simulink model "sampling_SH_lowpass_sinusoidal"  (R2020a)
settings: Solver=ode45  StartTime=0  StopTime=0.0504045  RelTol=1e-3  EnableMultiTasking=on
PreLoadFcn:
  | seed=123456789;
  | fs=100000;
libraries: dsparch4 x1, dspsigops x1
settings Model: Creator=morelos_zaragoza  LastModifiedBy=000098944
settings DataIOCC: LimitDataPoints=on  SaveFormat=Array  SignalLoggingSaveFormat=ModelDataLogs  ReturnWorkspaceOutputs=off
settings OptimizationCC: ExpressionDepthLimit=2147483647  InitFltsAndDblsToZero=on  LifeSpan=inf
settings DebuggingCC: SaveWithParameterizedLinksMsg=none  UnderspecifiedInitializationDetection=Classic  MergeDetectMultiDrivingBlocksExec=none  SignalResolutionControl=TryResolveAllWithWarning  SolverPrmCheckMsg=warning  MultiTaskDSMMsg=warning  MultiTaskCondExecSysMsg=none  FcnCallInpInsideContextMsg=warning  StateNameClashWarn=warning  SFUnexpectedBacktrackingDiag=warning  SFNoUnconditionalDefaultTransitionDiag=warning  SFExecutionAtInitializationDiag=none  ArithmeticOperatorsInVariantConditions=warning
settings HardwareCC: ProdBitPerPointer=32  ProdBitPerSizeT=32  ProdBitPerPtrDiffT=32  ProdLargestAtomicFloat=None  ProdIntDivRoundTo=Undefined  ProdEndianess=Unspecified  ProdWordSize=32  ProdHWDeviceType=32-bit Generic
settings ModelReferenceCC: PropagateSignalLabelsOutOfModel=off
settings SFSimCC: SimUseLocalCustomCode=off  CustomCodeUndefinedFunction=UseInterfaceOnly
settings RTWCC: RTWUseLocalCustomCode=off
settings CodeAppCC: StateflowObjectComments=on
settings GRTTargetCC: TargetFcnLib=ansi_tfl_tmw.mat  TargetLangStandard=C89/C90 (ANSI)  CombineOutputUpdateFcns=off  GRTInterface=on
settings ConfigComp: CovMetricSettings=dw  CovHtmlReporting=on  CovSaveCumulativeToWorkspaceVar=on  CovSaveSingleToWorkspaceVar=on  CovExternalEMLEnable=off

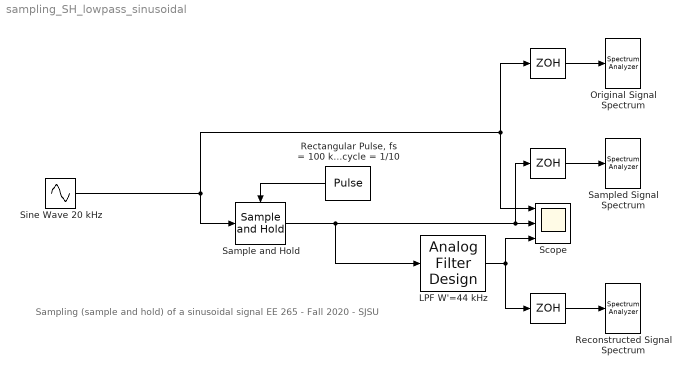
== system sampling_SH_lowpass_sinusoidal ==
  note: Sampling (sample and hold) of a sinusoidal signal
      | EE 265 - Fall 2020 - SJSU
  "  " : ZeroOrderHold  SampleTime=1/600000
  "    " : ZeroOrderHold  SampleTime=1/600000
  "     " : ZeroOrderHold  SampleTime=1/600000
  " Original Signal Spectrum" : SpectrumAnalyzer
  LPF W'=44 kHz : dsparch4/Analog Filter Design  method=Butterworth  filttype=Lowpass  N=8  Wlo=2*pi*44000  Whi=2*pi*110  Rp=2  Rs=40
  Reconstructed Signal Spectrum : SpectrumAnalyzer
  "Rectangular Pulse, fs = 100 kHz Duty cycle = 1/10" : DiscretePulseGenerator  PulseType=Time based  Period=1/fs  PulseWidth=10  SampleTime=1e-2/2)
  Sample and Hold : dspsigops/Sample and Hold  trig=Rising edge  initCond=0  latchinput=off
  Sampled Signal Spectrum : SpectrumAnalyzer
  Scope : Scope  NumInputPorts=3
  Sine Wave 20 kHz : Sin  Frequency=2*pi*20000  Phase=pi/6  SampleTime=0
  wires:
  Sample and Hold/1 -> LPF W'=44 kHz/1, "  "/1, Scope/2
  "  "/1 -> Sampled Signal Spectrum/1
  Sine Wave 20 kHz/1 -> Sample and Hold/1, "     "/1, Scope/1
  LPF W'=44 kHz/1 -> Scope/3, "    "/1
  "    "/1 -> Reconstructed Signal Spectrum/1
  "Rectangular Pulse, fs = 100 kHz Duty cycle = 1/10"/1 -> Sample and Hold/Trigger
  "     "/1 -> " Original Signal Spectrum"/1
